simulink model "drone_diagram"  (R2021a)
settings: Solver=VariableStepAuto  StartTime=0.0  StopTime=10.0  RelTol=1e-3
values from neighbouring files (symbols this model uses):
  air_density = 1.225    [hw3.m]
  J = [Jxx 0 0; 0 Jyy 0; 0 0 Jzz]    [hw3.m]
  m = 0.068    [hw3.m]
  offset = k_estimate(1)    [hw3.m]
  prop_diam = 0.066    [hw3.m]
  slope = k_estimate(2)    [hw3.m]
  x_dist = 0.047625    [hw3.m]
  y_dist = 0.047625    [hw3.m]
undefined symbols (not defined in the file or in its folder): u1
libraries: vrlib x2, aerolibutil x1
settings Model: Creator=willwu  LastModifiedBy=willwu

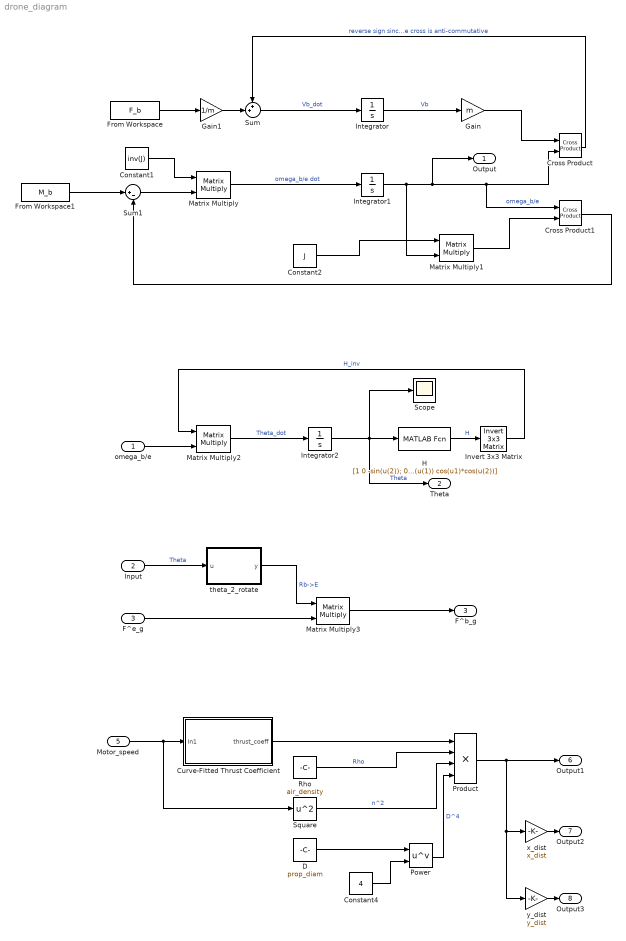
== system drone_diagram ==
  omega_b/e : Inport
  Input : Inport  Port=2
  F^e_g : Inport  Port=3
  Motor_speed : Inport  Port=5
  Constant1 : Constant  Value=inv(J)
  Constant2 : Constant  Value=J
  Constant4 : Constant  Value=4
  Cross Product : vrlib/Utilities/Cross Product
  Cross Product1 : vrlib/Utilities/Cross Product
  Curve-Fitted Thrust Coefficient : Subsystem
  D : Constant  Value=prop_diam
  From Workspace : FromWorkspace  VariableName=F_b
  From Workspace1 : FromWorkspace  VariableName=M_b
  Gain : Gain  Gain=m
  Gain1 : Gain  Gain=1/m
  H : MATLABFcn  MATLABFcn=[1 0 -sin(u(2)); 0 cos(u(1)) sin(u(1))*cos(u(2)); 0 -sin(u(1)) cos(u1)*cos(u(2))]  OutputDimensions=[3 3]  Output1D=off
  Integrator : Integrator
  Integrator1 : Integrator
  Integrator2 : Integrator
  Invert 3x3 Matrix : aerolibutil/Invert  3x3 Matrix
  Matrix Multiply{,1..3} (4 alike) : Product  Multiplication=Matrix(*)
  Power : Math  Operator=pow  SaturateOnIntegerOverflow=on
  Product : Product  Inputs=4
  Rho : Constant  Value=air_density
  Scope : Scope
  Square : Math  Operator=square  SaturateOnIntegerOverflow=on
  Sum : Sum  Inputs=++|
  Sum1 : Sum  Inputs=|+-
  theta_2_rotate : MATLAB Function  TreatAsAtomicUnit=on
  x_dist : Gain  Gain=x_dist
  y_dist : Gain  Gain=y_dist
  Output : Outport  SignalName=omega_b/e
  Theta : Outport  Port=2  SignalName=Theta
  F^b_g : Outport  Port=3  SignalName=F^b_g
  Output1 : Outport  Port=6  SignalName=Thrust
  Output2 : Outport  Port=7  SignalName=pitching_moment
  Output3 : Outport  Port=8  SignalName=rolling_moment
  wires:
  Sum/1 -> Integrator/1  "Vb_dot"
  Integrator/1 -> Gain/1  "Vb"
  Matrix Multiply/1 -> Integrator1/1  "omega_b/e dot"
  Integrator1/1 -> Matrix Multiply1/2, Output/1, Cross Product/2, Cross Product1/1  "omega_b/e"
  Cross Product/1 -> Sum/1  "reverse sign since cross is anti-commutative"
  Gain/1 -> Cross Product/1
  From Workspace/1 -> Gain1/1
  Gain1/1 -> Sum/2
  Constant1/1 -> Matrix Multiply/1
  Constant2/1 -> Matrix Multiply1/1
  Matrix Multiply1/1 -> Cross Product1/2
  Sum1/1 -> Matrix Multiply/2
  Cross Product1/1 -> Sum1/2
  From Workspace1/1 -> Sum1/1
  Integrator2/1 -> Theta/1, Scope/1, H/1  "Theta"
  Matrix Multiply2/1 -> Integrator2/1  "Theta_dot"
  H/1 -> Invert 3x3 Matrix/1  "H"
  Invert 3x3 Matrix/1 -> Matrix Multiply2/1  "H_inv"
  omega_b/e/1 -> Matrix Multiply2/2
  F^e_g/1 -> Matrix Multiply3/2
  Input/1 -> theta_2_rotate/1(u)  "Theta"
  theta_2_rotate/1(y) -> Matrix Multiply3/1  "Rb->E"
  Matrix Multiply3/1 -> F^b_g/1
  Motor_speed/1 -> Square/1, Curve-Fitted Thrust Coefficient/1(In1)
  Curve-Fitted Thrust Coefficient/1(thrust_coeff) -> Product/1
  Square/1 -> Product/3  "n^2"
  Rho/1 -> Product/2  "Rho"
  D/1 -> Power/1
  Product/1 -> y_dist/1, x_dist/1, Output1/1
  Constant4/1 -> Power/2
  Power/1 -> Product/4  "D^4"
  x_dist/1 -> Output2/1
  y_dist/1 -> Output3/1

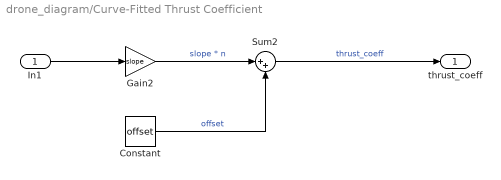
== system drone_diagram/Curve-Fitted Thrust Coefficient ==
  In1 : Inport
  Constant : Constant  Value=offset
  Gain2 : Gain  Gain=slope
  Sum2 : Sum  Inputs=|++
  thrust_coeff : Outport
  wires:
  Constant/1 -> Sum2/2  "offset"
  Gain2/1 -> Sum2/1  "slope * n"
  Sum2/1 -> thrust_coeff/1  "thrust_coeff"
  In1/1 -> Gain2/1

== matlab function drone_diagram/theta_2_rotate ==
  data: u input; y output
function y = fcn(u)
    phi = u(1);
    theta = u(2);
    psi = u(3);
    
    R_phi = [1 0 0;0 cos(phi) sin(phi); 0 -sin(phi) cos(phi)];
    R_theta = [cos(theta) 0 -sin(theta); 0 1 0; sin(theta) 0 cos(theta)];
    R_psi = [cos(psi) sin(psi) 0; -sin(psi) cos(psi) 0; 0 0 1];
    
y = R_phi * R_theta * R_psi;
